simulink model "final_model"  (R2023b)
settings: Solver=VariableStepAuto  StartTime=0.0  StopTime=200  RelTol=1e-3
(part 3 of 3)

== system final_model/40g ==
  " u(t)" : Inport
  p(t) : Inport  Port=2
  Constant : Constant  Value=p1*Gb
  Constant1 : Constant  Value=p1
  Gain : Gain  Gain=1/V
  Gain1 : Gain  Gain=n
  Gain2 : Gain  Gain=p3
  Gain3 : Gain  Gain=-p2
  Gain4 : Gain  Gain=1/V
  Integrator : Integrator
  Integrator1 : Integrator
  Integrator2 : Integrator  InitialCondition=G0
  Product : Product
  Sum : Sum  Inputs=|+-
  Sum1 : Sum  Inputs=|++
  Sum2 : Sum  Inputs=|++-
  Sum3 : Sum  Inputs=|++
  " G(t)" : Outport
  X(t) : Outport  Port=2
  I(t) : Outport  Port=3
  wires:
  " u(t)"/1 -> Gain/1
  Gain/1 -> Sum/1
  Sum/1 -> Integrator/1
  Integrator/1 -> Gain2/1, I(t)/1, Gain1/1
  Gain1/1 -> Sum/2
  Gain2/1 -> Sum1/1
  Gain3/1 -> Sum1/2
  Integrator1/1 -> Gain3/1, Sum3/2, X(t)/1
  p(t)/1 -> Gain4/1
  Gain4/1 -> Sum2/1
  Constant/1 -> Sum2/2
  Constant1/1 -> Sum3/1
  Sum2/1 -> Integrator2/1
  Product/1 -> Sum2/3
  Sum3/1 -> Product/2
  Integrator2/1 -> Product/1, " G(t)"/1
  Sum1/1 -> Integrator1/1

== system final_model/40g.1 ==
  " u(t)" : Inport
  p(t) : Inport  Port=2
  Constant : Constant  Value=p1*Gb
  Constant1 : Constant  Value=p1
  Gain : Gain  Gain=1/V
  Gain1 : Gain  Gain=n
  Gain2 : Gain  Gain=p3
  Gain3 : Gain  Gain=-p2
  Gain4 : Gain  Gain=1/V
  Integrator : Integrator
  Integrator1 : Integrator
  Integrator2 : Integrator  InitialCondition=G0
  Product : Product
  Sum : Sum  Inputs=|+-
  Sum1 : Sum  Inputs=|++
  Sum2 : Sum  Inputs=|++-
  Sum3 : Sum  Inputs=|++
  " G(t)" : Outport
  X(t) : Outport  Port=2
  I(t) : Outport  Port=3
  wires:
  " u(t)"/1 -> Gain/1
  Gain/1 -> Sum/1
  Sum/1 -> Integrator/1
  Integrator/1 -> Gain2/1, I(t)/1, Gain1/1
  Gain1/1 -> Sum/2
  Gain2/1 -> Sum1/1
  Gain3/1 -> Sum1/2
  Integrator1/1 -> Gain3/1, Sum3/2, X(t)/1
  p(t)/1 -> Gain4/1
  Gain4/1 -> Sum2/1
  Constant/1 -> Sum2/2
  Constant1/1 -> Sum3/1
  Sum2/1 -> Integrator2/1
  Product/1 -> Sum2/3
  Sum3/1 -> Product/2
  Integrator2/1 -> Product/1, " G(t)"/1
  Sum1/1 -> Integrator1/1

== system final_model/40g1 ==
  " u(t)" : Inport
  p(t) : Inport  Port=2
  Constant : Constant  Value=p1*Gb
  Constant1 : Constant  Value=p1
  Gain : Gain  Gain=1/V
  Gain1 : Gain  Gain=n
  Gain2 : Gain  Gain=p3
  Gain3 : Gain  Gain=-p2
  Gain4 : Gain  Gain=1/V
  Integrator : Integrator
  Integrator1 : Integrator
  Integrator2 : Integrator  InitialCondition=G0
  Product : Product
  Sum : Sum  Inputs=|+-
  Sum1 : Sum  Inputs=|++
  Sum2 : Sum  Inputs=|++-
  Sum3 : Sum  Inputs=|++
  " G(t)" : Outport
  X(t) : Outport  Port=2
  I(t) : Outport  Port=3
  wires:
  " u(t)"/1 -> Gain/1
  Gain/1 -> Sum/1
  Sum/1 -> Integrator/1
  Integrator/1 -> Gain2/1, I(t)/1, Gain1/1
  Gain1/1 -> Sum/2
  Gain2/1 -> Sum1/1
  Gain3/1 -> Sum1/2
  Integrator1/1 -> Gain3/1, Sum3/2, X(t)/1
  p(t)/1 -> Gain4/1
  Gain4/1 -> Sum2/1
  Constant/1 -> Sum2/2
  Constant1/1 -> Sum3/1
  Sum2/1 -> Integrator2/1
  Product/1 -> Sum2/3
  Sum3/1 -> Product/2
  Integrator2/1 -> Product/1, " G(t)"/1
  Sum1/1 -> Integrator1/1

== system final_model/70.1g ==
  p(t) : Inport
  u(t) : Inport  Port=2
  Constant : Constant  Value=Gb
  Constant1 : Constant  Value=p1
  Gain : Gain  Gain=1/V
  Gain1 : Gain  Gain=p1
  Gain2 : Gain  Gain=p2
  Gain3 : Gain  Gain=1/V
  Gain4 : Gain  Gain=n
  Gain5 : Gain  Gain=p3
  Integrator : Integrator  InitialCondition=G0
  Integrator1 : Integrator
  Integrator2 : Integrator
  Product : Product
  Product1 : Product
  Sum : Sum  Inputs=|++--
  Sum1 : Sum  Inputs=|+-
  Sum2 : Sum  Inputs=|+-
  G(t) : Outport
  X(t) : Outport  Port=2
  I(t) : Outport  Port=3
  wires:
  Sum2/1 -> Integrator2/1
  Gain3/1 -> Sum2/1
  Sum1/1 -> Integrator1/1
  Integrator2/1 -> Gain4/1, I(t)/1, Gain5/1
  u(t)/1 -> Gain3/1
  Integrator1/1 -> Product1/2, X(t)/1, Gain2/1
  Product/1 -> Sum/2
  Integrator/1 -> G(t)/1, Gain1/1, Product1/1
  Gain5/1 -> Sum1/1
  Sum/1 -> Integrator/1
  Constant1/1 -> Product/2
  Constant/1 -> Product/1
  Gain4/1 -> Sum2/2
  Gain2/1 -> Sum1/2
  Product1/1 -> Sum/3
  Gain1/1 -> Sum/4
  p(t)/1 -> Gain/1
  Gain/1 -> Sum/1

== system final_model/70.1g1 ==
  p(t) : Inport
  u(t) : Inport  Port=2
  Constant : Constant  Value=Gb
  Constant1 : Constant  Value=p1
  Gain : Gain  Gain=1/V
  Gain1 : Gain  Gain=p1
  Gain2 : Gain  Gain=p2
  Gain3 : Gain  Gain=1/V
  Gain4 : Gain  Gain=n
  Gain5 : Gain  Gain=p3
  Integrator : Integrator  InitialCondition=G0
  Integrator1 : Integrator
  Integrator2 : Integrator
  Product : Product
  Product1 : Product
  Sum : Sum  Inputs=|++--
  Sum1 : Sum  Inputs=|+-
  Sum2 : Sum  Inputs=|+-
  G(t) : Outport
  X(t) : Outport  Port=2
  I(t) : Outport  Port=3
  wires:
  Sum2/1 -> Integrator2/1
  Gain3/1 -> Sum2/1
  Sum1/1 -> Integrator1/1
  Integrator2/1 -> Gain4/1, I(t)/1, Gain5/1
  u(t)/1 -> Gain3/1
  Integrator1/1 -> Product1/2, X(t)/1, Gain2/1
  Product/1 -> Sum/2
  Integrator/1 -> G(t)/1, Gain1/1, Product1/1
  Gain5/1 -> Sum1/1
  Sum/1 -> Integrator/1
  Constant1/1 -> Product/2
  Constant/1 -> Product/1
  Gain4/1 -> Sum2/2
  Gain2/1 -> Sum1/2
  Product1/1 -> Sum/3
  Gain1/1 -> Sum/4
  p(t)/1 -> Gain/1
  Gain/1 -> Sum/1

== system final_model/70g ==
  " u(t)" : Inport
  p(t) : Inport  Port=2
  Constant : Constant  Value=p1*Gb
  Constant1 : Constant  Value=p1
  Gain : Gain  Gain=1/V
  Gain1 : Gain  Gain=n
  Gain2 : Gain  Gain=p3
  Gain3 : Gain  Gain=-p2
  Gain4 : Gain  Gain=1/V
  Integrator : Integrator
  Integrator1 : Integrator
  Integrator2 : Integrator  InitialCondition=G0
  Product : Product
  Sum : Sum  Inputs=|+-
  Sum1 : Sum  Inputs=|++
  Sum2 : Sum  Inputs=|++-
  Sum3 : Sum  Inputs=|++
  " G(t)" : Outport
  X(t) : Outport  Port=2
  I(t) : Outport  Port=3
  wires:
  " u(t)"/1 -> Gain/1
  Gain/1 -> Sum/1
  Sum/1 -> Integrator/1
  Integrator/1 -> Gain2/1, I(t)/1, Gain1/1
  Gain1/1 -> Sum/2
  Gain2/1 -> Sum1/1
  Gain3/1 -> Sum1/2
  Integrator1/1 -> Gain3/1, Sum3/2, X(t)/1
  p(t)/1 -> Gain4/1
  Gain4/1 -> Sum2/1
  Constant/1 -> Sum2/2
  Constant1/1 -> Sum3/1
  Sum2/1 -> Integrator2/1
  Product/1 -> Sum2/3
  Sum3/1 -> Product/2
  Integrator2/1 -> Product/1, " G(t)"/1
  Sum1/1 -> Integrator1/1

== system final_model/70g.1 ==
  " u(t)" : Inport
  p(t) : Inport  Port=2
  Constant : Constant  Value=p1*Gb
  Constant1 : Constant  Value=p1
  Gain : Gain  Gain=1/V
  Gain1 : Gain  Gain=n
  Gain2 : Gain  Gain=p3
  Gain3 : Gain  Gain=-p2
  Gain4 : Gain  Gain=1/V
  Integrator : Integrator
  Integrator1 : Integrator
  Integrator2 : Integrator  InitialCondition=G0
  Product : Product
  Sum : Sum  Inputs=|+-
  Sum1 : Sum  Inputs=|++
  Sum2 : Sum  Inputs=|++-
  Sum3 : Sum  Inputs=|++
  " G(t)" : Outport
  X(t) : Outport  Port=2
  I(t) : Outport  Port=3
  wires:
  " u(t)"/1 -> Gain/1
  Gain/1 -> Sum/1
  Sum/1 -> Integrator/1
  Integrator/1 -> Gain2/1, I(t)/1, Gain1/1
  Gain1/1 -> Sum/2
  Gain2/1 -> Sum1/1
  Gain3/1 -> Sum1/2
  Integrator1/1 -> Gain3/1, Sum3/2, X(t)/1
  p(t)/1 -> Gain4/1
  Gain4/1 -> Sum2/1
  Constant/1 -> Sum2/2
  Constant1/1 -> Sum3/1
  Sum2/1 -> Integrator2/1
  Product/1 -> Sum2/3
  Sum3/1 -> Product/2
  Integrator2/1 -> Product/1, " G(t)"/1
  Sum1/1 -> Integrator1/1

== system final_model/70g1 ==
  " u(t)" : Inport
  p(t) : Inport  Port=2
  Constant : Constant  Value=p1*Gb
  Constant1 : Constant  Value=p1
  Gain : Gain  Gain=1/V
  Gain1 : Gain  Gain=n
  Gain2 : Gain  Gain=p3
  Gain3 : Gain  Gain=-p2
  Gain4 : Gain  Gain=1/V
  Integrator : Integrator
  Integrator1 : Integrator
  Integrator2 : Integrator  InitialCondition=G0
  Product : Product
  Sum : Sum  Inputs=|+-
  Sum1 : Sum  Inputs=|++
  Sum2 : Sum  Inputs=|++-
  Sum3 : Sum  Inputs=|++
  " G(t)" : Outport
  X(t) : Outport  Port=2
  I(t) : Outport  Port=3
  wires:
  " u(t)"/1 -> Gain/1
  Gain/1 -> Sum/1
  Sum/1 -> Integrator/1
  Integrator/1 -> Gain2/1, I(t)/1, Gain1/1
  Gain1/1 -> Sum/2
  Gain2/1 -> Sum1/1
  Gain3/1 -> Sum1/2
  Integrator1/1 -> Gain3/1, Sum3/2, X(t)/1
  p(t)/1 -> Gain4/1
  Gain4/1 -> Sum2/1
  Constant/1 -> Sum2/2
  Constant1/1 -> Sum3/1
  Sum2/1 -> Integrator2/1
  Product/1 -> Sum2/3
  Sum3/1 -> Product/2
  Integrator2/1 -> Product/1, " G(t)"/1
  Sum1/1 -> Integrator1/1

== system final_model/DG 100g ==
  " u(t)" : Inport
  p(t) : Inport  Port=2
  Constant : Constant  Value=p1*Gb
  Constant1 : Constant  Value=p1
  Gain : Gain  Gain=1/V
  Gain1 : Gain  Gain=n
  Gain2 : Gain  Gain=p3
  Gain3 : Gain  Gain=-p2
  Gain4 : Gain  Gain=1/V
  Integrator : Integrator
  Integrator1 : Integrator
  Integrator2 : Integrator  InitialCondition=G0
  Product : Product
  Sum : Sum  Inputs=|+-
  Sum1 : Sum  Inputs=|++
  Sum2 : Sum  Inputs=|++-
  Sum3 : Sum  Inputs=|++
  " G(t)" : Outport
  X(t) : Outport  Port=2
  I(t) : Outport  Port=3
  wires:
  " u(t)"/1 -> Gain/1
  Gain/1 -> Sum/1
  Sum/1 -> Integrator/1
  Integrator/1 -> Gain2/1, I(t)/1, Gain1/1
  Gain1/1 -> Sum/2
  Gain2/1 -> Sum1/1
  Gain3/1 -> Sum1/2
  Integrator1/1 -> Gain3/1, Sum3/2, X(t)/1
  p(t)/1 -> Gain4/1
  Gain4/1 -> Sum2/1
  Constant/1 -> Sum2/2
  Constant1/1 -> Sum3/1
  Sum2/1 -> Integrator2/1
  Product/1 -> Sum2/3
  Sum3/1 -> Product/2
  Integrator2/1 -> Product/1, " G(t)"/1
  Sum1/1 -> Integrator1/1

== system final_model/DG 10g ==
  " u(t)" : Inport
  p(t) : Inport  Port=2
  Constant : Constant  Value=p1*Gb
  Constant1 : Constant  Value=p1
  Gain : Gain  Gain=1/V
  Gain1 : Gain  Gain=n
  Gain2 : Gain  Gain=p3
  Gain3 : Gain  Gain=-p2
  Gain4 : Gain  Gain=1/V
  Integrator : Integrator
  Integrator1 : Integrator
  Integrator2 : Integrator  InitialCondition=G0
  Product : Product
  Sum : Sum  Inputs=|+-
  Sum1 : Sum  Inputs=|++
  Sum2 : Sum  Inputs=|++-
  Sum3 : Sum  Inputs=|++
  " G(t)" : Outport
  X(t) : Outport  Port=2
  I(t) : Outport  Port=3
  wires:
  " u(t)"/1 -> Gain/1
  Gain/1 -> Sum/1
  Sum/1 -> Integrator/1
  Integrator/1 -> Gain2/1, I(t)/1, Gain1/1
  Gain1/1 -> Sum/2
  Gain2/1 -> Sum1/1
  Gain3/1 -> Sum1/2
  Integrator1/1 -> Gain3/1, Sum3/2, X(t)/1
  p(t)/1 -> Gain4/1
  Gain4/1 -> Sum2/1
  Constant/1 -> Sum2/2
  Constant1/1 -> Sum3/1
  Sum2/1 -> Integrator2/1
  Product/1 -> Sum2/3
  Sum3/1 -> Product/2
  Integrator2/1 -> Product/1, " G(t)"/1
  Sum1/1 -> Integrator1/1

== system final_model/DG 40g ==
  " u(t)" : Inport
  p(t) : Inport  Port=2
  Constant : Constant  Value=p1*Gb
  Constant1 : Constant  Value=p1
  Gain : Gain  Gain=1/V
  Gain1 : Gain  Gain=n
  Gain2 : Gain  Gain=p3
  Gain3 : Gain  Gain=-p2
  Gain4 : Gain  Gain=1/V
  Integrator : Integrator
  Integrator1 : Integrator
  Integrator2 : Integrator  InitialCondition=G0
  Product : Product
  Sum : Sum  Inputs=|+-
  Sum1 : Sum  Inputs=|++
  Sum2 : Sum  Inputs=|++-
  Sum3 : Sum  Inputs=|++
  " G(t)" : Outport
  X(t) : Outport  Port=2
  I(t) : Outport  Port=3
  wires:
  " u(t)"/1 -> Gain/1
  Gain/1 -> Sum/1
  Sum/1 -> Integrator/1
  Integrator/1 -> Gain2/1, I(t)/1, Gain1/1
  Gain1/1 -> Sum/2
  Gain2/1 -> Sum1/1
  Gain3/1 -> Sum1/2
  Integrator1/1 -> Gain3/1, Sum3/2, X(t)/1
  p(t)/1 -> Gain4/1
  Gain4/1 -> Sum2/1
  Constant/1 -> Sum2/2
  Constant1/1 -> Sum3/1
  Sum2/1 -> Integrator2/1
  Product/1 -> Sum2/3
  Sum3/1 -> Product/2
  Integrator2/1 -> Product/1, " G(t)"/1
  Sum1/1 -> Integrator1/1

== system final_model/DG 70g ==
  " u(t)" : Inport
  p(t) : Inport  Port=2
  Constant : Constant  Value=p1*Gb
  Constant1 : Constant  Value=p1
  Gain : Gain  Gain=1/V
  Gain1 : Gain  Gain=n
  Gain2 : Gain  Gain=p3
  Gain3 : Gain  Gain=-p2
  Gain4 : Gain  Gain=1/V
  Integrator : Integrator
  Integrator1 : Integrator
  Integrator2 : Integrator  InitialCondition=G0
  Product : Product
  Sum : Sum  Inputs=|+-
  Sum1 : Sum  Inputs=|++
  Sum2 : Sum  Inputs=|++-
  Sum3 : Sum  Inputs=|++
  " G(t)" : Outport
  X(t) : Outport  Port=2
  I(t) : Outport  Port=3
  wires:
  " u(t)"/1 -> Gain/1
  Gain/1 -> Sum/1
  Sum/1 -> Integrator/1
  Integrator/1 -> Gain2/1, I(t)/1, Gain1/1
  Gain1/1 -> Sum/2
  Gain2/1 -> Sum1/1
  Gain3/1 -> Sum1/2
  Integrator1/1 -> Gain3/1, Sum3/2, X(t)/1
  p(t)/1 -> Gain4/1
  Gain4/1 -> Sum2/1
  Constant/1 -> Sum2/2
  Constant1/1 -> Sum3/1
  Sum2/1 -> Integrator2/1
  Product/1 -> Sum2/3
  Sum3/1 -> Product/2
  Integrator2/1 -> Product/1, " G(t)"/1
  Sum1/1 -> Integrator1/1

== system final_model/model liniar1 ==
  p(t) : Inport
  u(t) : Inport  Port=2
  Constant : Constant  Value=Gb
  Gain : Gain  Gain=1/V
  Gain1 : Gain  Gain=p1
  Gain2 : Gain  Gain=p2
  Gain3 : Gain  Gain=1/V
  Gain4 : Gain  Gain=n
  Gain5 : Gain  Gain=p3
  Integrator : Integrator  InitialCondition=G0
  Integrator1 : Integrator
  Integrator2 : Integrator
  Product : Product
  Product1 : Product
  Sum : Sum  Inputs=|+---
  Sum1 : Sum  Inputs=|+-
  Sum2 : Sum  Inputs=|+-
  Xb : Constant  Value=Xb
  G(t) : Outport
  X(t) : Outport  Port=2
  I(t) : Outport  Port=3
  wires:
  p(t)/1 -> Gain/1
  Gain/1 -> Sum/1
  Constant/1 -> Product/1
  Product/1 -> Sum/2
  Sum/1 -> Integrator/1
  Integrator/1 -> Gain1/1, Product1/1, G(t)/1
  Xb/1 -> Product1/2
  Product1/1 -> Sum/3
  Gain1/1 -> Sum/4
  Integrator1/1 -> Product/2, X(t)/1, Gain2/1
  Gain2/1 -> Sum1/2
  Integrator2/1 -> Gain4/1, I(t)/1, Gain5/1
  Sum2/1 -> Integrator2/1
  Gain5/1 -> Sum1/1
  Gain4/1 -> Sum2/2
  u(t)/1 -> Gain3/1
  Gain3/1 -> Sum2/1
  Sum1/1 -> Integrator1/1

== system final_model/model liniar2 ==
  p(t) : Inport
  u(t) : Inport  Port=2
  Constant : Constant  Value=Gb
  Gain : Gain  Gain=1/V
  Gain1 : Gain  Gain=p1
  Gain2 : Gain  Gain=p2
  Gain3 : Gain  Gain=1/V
  Gain4 : Gain  Gain=n
  Gain5 : Gain  Gain=p3
  Integrator : Integrator  InitialCondition=G0
  Integrator1 : Integrator
  Integrator2 : Integrator
  Product : Product
  Product1 : Product
  Sum : Sum  Inputs=|+---
  Sum1 : Sum  Inputs=|+-
  Sum2 : Sum  Inputs=|+-
  Xb : Constant  Value=Xb
  G(t) : Outport
  X(t) : Outport  Port=2
  I(t) : Outport  Port=3
  wires:
  p(t)/1 -> Gain/1
  Gain/1 -> Sum/1
  Constant/1 -> Product/1
  Product/1 -> Sum/2
  Sum/1 -> Integrator/1
  Integrator/1 -> Gain1/1, Product1/1, G(t)/1
  Xb/1 -> Product1/2
  Product1/1 -> Sum/3
  Gain1/1 -> Sum/4
  Integrator1/1 -> Product/2, X(t)/1, Gain2/1
  Gain2/1 -> Sum1/2
  Integrator2/1 -> Gain4/1, I(t)/1, Gain5/1
  Sum2/1 -> Integrator2/1
  Gain5/1 -> Sum1/1
  Gain4/1 -> Sum2/2
  u(t)/1 -> Gain3/1
  Gain3/1 -> Sum2/1
  Sum1/1 -> Integrator1/1

== system final_model/model liniar3 ==
  p(t) : Inport
  u(t) : Inport  Port=2
  Constant : Constant  Value=Gb
  Gain : Gain  Gain=1/V
  Gain1 : Gain  Gain=p1
  Gain2 : Gain  Gain=p2
  Gain3 : Gain  Gain=1/V
  Gain4 : Gain  Gain=n
  Gain5 : Gain  Gain=p3
  Integrator : Integrator  InitialCondition=G0
  Integrator1 : Integrator
  Integrator2 : Integrator
  Product : Product
  Product1 : Product
  Sum : Sum  Inputs=|+---
  Sum1 : Sum  Inputs=|+-
  Sum2 : Sum  Inputs=|+-
  Xb : Constant  Value=Xb
  G(t) : Outport
  X(t) : Outport  Port=2
  I(t) : Outport  Port=3
  wires:
  p(t)/1 -> Gain/1
  Gain/1 -> Sum/1
  Constant/1 -> Product/1
  Product/1 -> Sum/2
  Sum/1 -> Integrator/1
  Integrator/1 -> Gain1/1, Product1/1, G(t)/1
  Xb/1 -> Product1/2
  Product1/1 -> Sum/3
  Gain1/1 -> Sum/4
  Integrator1/1 -> Product/2, X(t)/1, Gain2/1
  Gain2/1 -> Sum1/2
  Integrator2/1 -> Gain4/1, I(t)/1, Gain5/1
  Sum2/1 -> Integrator2/1
  Gain5/1 -> Sum1/1
  Gain4/1 -> Sum2/2
  u(t)/1 -> Gain3/1
  Gain3/1 -> Sum2/1
  Sum1/1 -> Integrator1/1

== system final_model/model liniar4 ==
  p(t) : Inport
  u(t) : Inport  Port=2
  Constant : Constant  Value=Gb
  Gain : Gain  Gain=1/V
  Gain1 : Gain  Gain=p1
  Gain2 : Gain  Gain=p2
  Gain3 : Gain  Gain=1/V
  Gain4 : Gain  Gain=n
  Gain5 : Gain  Gain=p3
  Integrator : Integrator  InitialCondition=G0
  Integrator1 : Integrator
  Integrator2 : Integrator
  Product : Product
  Product1 : Product
  Sum : Sum  Inputs=|+---
  Sum1 : Sum  Inputs=|+-
  Sum2 : Sum  Inputs=|+-
  Xb : Constant  Value=Xb
  G(t) : Outport
  X(t) : Outport  Port=2
  I(t) : Outport  Port=3
  wires:
  p(t)/1 -> Gain/1
  Gain/1 -> Sum/1
  Constant/1 -> Product/1
  Product/1 -> Sum/2
  Sum/1 -> Integrator/1
  Integrator/1 -> Gain1/1, Product1/1, G(t)/1
  Xb/1 -> Product1/2
  Product1/1 -> Sum/3
  Gain1/1 -> Sum/4
  Integrator1/1 -> Product/2, X(t)/1, Gain2/1
  Gain2/1 -> Sum1/2
  Integrator2/1 -> Gain4/1, I(t)/1, Gain5/1
  Sum2/1 -> Integrator2/1
  Gain5/1 -> Sum1/1
  Gain4/1 -> Sum2/2
  u(t)/1 -> Gain3/1
  Gain3/1 -> Sum2/1
  Sum1/1 -> Integrator1/1

== system final_model/model_neliniar1 ==
  p(t) : Inport
  u(t) : Inport  Port=2
  Constant : Constant  Value=Gb
  Constant1 : Constant  Value=p1
  Gain : Gain  Gain=1/V
  Gain1 : Gain  Gain=p1
  Gain2 : Gain  Gain=p2
  Gain3 : Gain  Gain=1/V
  Gain4 : Gain  Gain=n
  Gain5 : Gain  Gain=p3
  Integrator : Integrator  InitialCondition=G0
  Integrator1 : Integrator
  Integrator2 : Integrator
  Product : Product
  Product1 : Product
  Sum : Sum  Inputs=|++--
  Sum1 : Sum  Inputs=|+-
  Sum2 : Sum  Inputs=|+-
  G(t) : Outport
  X(t) : Outport  Port=2
  I(t) : Outport  Port=3
  wires:
  Sum2/1 -> Integrator2/1
  Gain3/1 -> Sum2/1
  Sum1/1 -> Integrator1/1
  Integrator2/1 -> Gain4/1, I(t)/1, Gain5/1
  u(t)/1 -> Gain3/1
  Integrator1/1 -> Product1/2, X(t)/1, Gain2/1
  Product/1 -> Sum/2
  Integrator/1 -> G(t)/1, Gain1/1, Product1/1
  Gain5/1 -> Sum1/1
  Sum/1 -> Integrator/1
  Constant1/1 -> Product/2
  Constant/1 -> Product/1
  Gain4/1 -> Sum2/2
  Gain2/1 -> Sum1/2
  Product1/1 -> Sum/3
  Gain1/1 -> Sum/4
  p(t)/1 -> Gain/1
  Gain/1 -> Sum/1

== system final_model/model_neliniar2 ==
  p(t) : Inport
  u(t) : Inport  Port=2
  Constant : Constant  Value=Gb
  Constant1 : Constant  Value=p1
  Gain : Gain  Gain=1/V
  Gain1 : Gain  Gain=p1
  Gain2 : Gain  Gain=p2
  Gain3 : Gain  Gain=1/V
  Gain4 : Gain  Gain=n
  Gain5 : Gain  Gain=p3
  Integrator : Integrator  InitialCondition=G0
  Integrator1 : Integrator
  Integrator2 : Integrator
  Product : Product
  Product1 : Product
  Sum : Sum  Inputs=|++--
  Sum1 : Sum  Inputs=|+-
  Sum2 : Sum  Inputs=|+-
  G(t) : Outport
  X(t) : Outport  Port=2
  I(t) : Outport  Port=3
  wires:
  Sum2/1 -> Integrator2/1
  Gain3/1 -> Sum2/1
  Sum1/1 -> Integrator1/1
  Integrator2/1 -> Gain4/1, I(t)/1, Gain5/1
  u(t)/1 -> Gain3/1
  Integrator1/1 -> Product1/2, X(t)/1, Gain2/1
  Product/1 -> Sum/2
  Integrator/1 -> G(t)/1, Gain1/1, Product1/1
  Gain5/1 -> Sum1/1
  Sum/1 -> Integrator/1
  Constant1/1 -> Product/2
  Constant/1 -> Product/1
  Gain4/1 -> Sum2/2
  Gain2/1 -> Sum1/2
  Product1/1 -> Sum/3
  Gain1/1 -> Sum/4
  p(t)/1 -> Gain/1
  Gain/1 -> Sum/1

== system final_model/model_neliniar3 ==
  p(t) : Inport
  u(t) : Inport  Port=2
  Constant : Constant  Value=Gb
  Constant1 : Constant  Value=p1
  Gain : Gain  Gain=1/V
  Gain1 : Gain  Gain=p1
  Gain2 : Gain  Gain=p2
  Gain3 : Gain  Gain=1/V
  Gain4 : Gain  Gain=n
  Gain5 : Gain  Gain=p3
  Integrator : Integrator  InitialCondition=G0
  Integrator1 : Integrator
  Integrator2 : Integrator
  Product : Product
  Product1 : Product
  Sum : Sum  Inputs=|++--
  Sum1 : Sum  Inputs=|+-
  Sum2 : Sum  Inputs=|+-
  G(t) : Outport
  X(t) : Outport  Port=2
  I(t) : Outport  Port=3
  wires:
  Sum2/1 -> Integrator2/1
  Gain3/1 -> Sum2/1
  Sum1/1 -> Integrator1/1
  Integrator2/1 -> Gain4/1, I(t)/1, Gain5/1
  u(t)/1 -> Gain3/1
  Integrator1/1 -> Product1/2, X(t)/1, Gain2/1
  Product/1 -> Sum/2
  Integrator/1 -> G(t)/1, Gain1/1, Product1/1
  Gain5/1 -> Sum1/1
  Sum/1 -> Integrator/1
  Constant1/1 -> Product/2
  Constant/1 -> Product/1
  Gain4/1 -> Sum2/2
  Gain2/1 -> Sum1/2
  Product1/1 -> Sum/3
  Gain1/1 -> Sum/4
  p(t)/1 -> Gain/1
  Gain/1 -> Sum/1

== system final_model/model_neliniar4 ==
  p(t) : Inport
  u(t) : Inport  Port=2
  Constant : Constant  Value=Gb
  Constant1 : Constant  Value=p1
  Gain : Gain  Gain=1/V
  Gain1 : Gain  Gain=p1
  Gain2 : Gain  Gain=p2
  Gain3 : Gain  Gain=1/V
  Gain4 : Gain  Gain=n
  Gain5 : Gain  Gain=p3
  Integrator : Integrator  InitialCondition=G0
  Integrator1 : Integrator
  Integrator2 : Integrator
  Product : Product
  Product1 : Product
  Sum : Sum  Inputs=|++--
  Sum1 : Sum  Inputs=|+-
  Sum2 : Sum  Inputs=|+-
  G(t) : Outport
  X(t) : Outport  Port=2
  I(t) : Outport  Port=3
  wires:
  Sum2/1 -> Integrator2/1
  Gain3/1 -> Sum2/1
  Sum1/1 -> Integrator1/1
  Integrator2/1 -> Gain4/1, I(t)/1, Gain5/1
  u(t)/1 -> Gain3/1
  Integrator1/1 -> Product1/2, X(t)/1, Gain2/1
  Product/1 -> Sum/2
  Integrator/1 -> G(t)/1, Gain1/1, Product1/1
  Gain5/1 -> Sum1/1
  Sum/1 -> Integrator/1
  Constant1/1 -> Product/2
  Constant/1 -> Product/1
  Gain4/1 -> Sum2/2
  Gain2/1 -> Sum1/2
  Product1/1 -> Sum/3
  Gain1/1 -> Sum/4
  p(t)/1 -> Gain/1
  Gain/1 -> Sum/1

== system final_model/perturbatie1 ==
  Clock : Clock
  Constant : Constant  Value=Dg
  Constant1 : Constant  Value=Ag
  Gain : Gain  Gain=-1/tg_max
  Gain1 : Gain  Gain=1/(tg_max*tg_max)
  Math Function : Math
  Product : Product  Inputs=4
  p(t) : Outport
  wires:
  Constant/1 -> Product/1
  Constant1/1 -> Product/2
  Clock/1 -> Gain/1, Product/3
  Gain/1 -> Math Function/1
  Math Function/1 -> Product/4
  Product/1 -> Gain1/1
  Gain1/1 -> p(t)/1

== system final_model/perturbatie10 ==
  Clock : Clock
  Constant : Constant  Value=Dg
  Constant1 : Constant  Value=Ag
  Gain : Gain  Gain=-1/tg_max
  Gain1 : Gain  Gain=1/(tg_max*tg_max)
  Math Function : Math
  Product : Product  Inputs=4
  p(t) : Outport
  wires:
  Constant/1 -> Product/1
  Constant1/1 -> Product/2
  Clock/1 -> Gain/1, Product/3
  Gain/1 -> Math Function/1
  Math Function/1 -> Product/4
  Product/1 -> Gain1/1
  Gain1/1 -> p(t)/1

== system final_model/perturbatie11 ==
  Clock : Clock
  Constant : Constant  Value=Dg
  Constant1 : Constant  Value=Ag
  Gain : Gain  Gain=-1/tg_max
  Gain1 : Gain  Gain=1/(tg_max*tg_max)
  Math Function : Math
  Product : Product  Inputs=4
  p(t) : Outport
  wires:
  Constant/1 -> Product/1
  Constant1/1 -> Product/2
  Clock/1 -> Gain/1, Product/3
  Gain/1 -> Math Function/1
  Math Function/1 -> Product/4
  Product/1 -> Gain1/1
  Gain1/1 -> p(t)/1

== system final_model/perturbatie12 ==
  Clock : Clock
  Constant : Constant  Value=Dg
  Constant1 : Constant  Value=Ag
  Gain : Gain  Gain=-1/tg_max
  Gain1 : Gain  Gain=1/(tg_max*tg_max)
  Math Function : Math
  Product : Product  Inputs=4
  p(t) : Outport
  wires:
  Constant/1 -> Product/1
  Constant1/1 -> Product/2
  Clock/1 -> Gain/1, Product/3
  Gain/1 -> Math Function/1
  Math Function/1 -> Product/4
  Product/1 -> Gain1/1
  Gain1/1 -> p(t)/1

== system final_model/perturbatie13 ==
  Clock : Clock
  Constant : Constant  Value=Dg
  Constant1 : Constant  Value=Ag
  Gain : Gain  Gain=-1/tg_max
  Gain1 : Gain  Gain=1/(tg_max*tg_max)
  Math Function : Math
  Product : Product  Inputs=4
  p(t) : Outport
  wires:
  Constant/1 -> Product/1
  Constant1/1 -> Product/2
  Clock/1 -> Gain/1, Product/3
  Gain/1 -> Math Function/1
  Math Function/1 -> Product/4
  Product/1 -> Gain1/1
  Gain1/1 -> p(t)/1

== system final_model/perturbatie15 ==
  Clock : Clock
  Constant : Constant  Value=Dg
  Constant1 : Constant  Value=Ag
  Gain : Gain  Gain=-1/tg_max
  Gain1 : Gain  Gain=1/(tg_max*tg_max)
  Math Function : Math
  Product : Product  Inputs=4
  p(t) : Outport
  wires:
  Constant/1 -> Product/1
  Constant1/1 -> Product/2
  Clock/1 -> Gain/1, Product/3
  Gain/1 -> Math Function/1
  Math Function/1 -> Product/4
  Product/1 -> Gain1/1
  Gain1/1 -> p(t)/1

== system final_model/perturbatie16 ==
  Clock : Clock
  Constant : Constant  Value=Dg
  Constant1 : Constant  Value=Ag
  Gain : Gain  Gain=-1/tg_max
  Gain1 : Gain  Gain=1/(tg_max*tg_max)
  Math Function : Math
  Product : Product  Inputs=4
  p(t) : Outport
  wires:
  Constant/1 -> Product/1
  Constant1/1 -> Product/2
  Clock/1 -> Gain/1, Product/3
  Gain/1 -> Math Function/1
  Math Function/1 -> Product/4
  Product/1 -> Gain1/1
  Gain1/1 -> p(t)/1

== system final_model/perturbatie17 ==
  Clock : Clock
  Constant : Constant  Value=Dg
  Constant1 : Constant  Value=Ag
  Gain : Gain  Gain=-1/tg_max
  Gain1 : Gain  Gain=1/(tg_max*tg_max)
  Math Function : Math
  Product : Product  Inputs=4
  p(t) : Outport
  wires:
  Constant/1 -> Product/1
  Constant1/1 -> Product/2
  Clock/1 -> Gain/1, Product/3
  Gain/1 -> Math Function/1
  Math Function/1 -> Product/4
  Product/1 -> Gain1/1
  Gain1/1 -> p(t)/1

== system final_model/perturbatie18 ==
  Clock : Clock
  Constant : Constant  Value=Dg
  Constant1 : Constant  Value=Ag
  Gain : Gain  Gain=-1/tg_max
  Gain1 : Gain  Gain=1/(tg_max*tg_max)
  Math Function : Math
  Product : Product  Inputs=4
  p(t) : Outport
  wires:
  Constant/1 -> Product/1
  Constant1/1 -> Product/2
  Clock/1 -> Gain/1, Product/3
  Gain/1 -> Math Function/1
  Math Function/1 -> Product/4
  Product/1 -> Gain1/1
  Gain1/1 -> p(t)/1

== system final_model/perturbatie19 ==
  Clock : Clock
  Constant : Constant  Value=Dg
  Constant1 : Constant  Value=Ag
  Gain : Gain  Gain=-1/tg_max
  Gain1 : Gain  Gain=1/(tg_max*tg_max)
  Math Function : Math
  Product : Product  Inputs=4
  p(t) : Outport
  wires:
  Constant/1 -> Product/1
  Constant1/1 -> Product/2
  Clock/1 -> Gain/1, Product/3
  Gain/1 -> Math Function/1
  Math Function/1 -> Product/4
  Product/1 -> Gain1/1
  Gain1/1 -> p(t)/1

== system final_model/perturbatie2 ==
  Clock : Clock
  Constant : Constant  Value=Dg
  Constant1 : Constant  Value=Ag
  Gain : Gain  Gain=-1/tg_max
  Gain1 : Gain  Gain=1/(tg_max*tg_max)
  Math Function : Math
  Product : Product  Inputs=4
  p(t) : Outport
  wires:
  Constant/1 -> Product/1
  Constant1/1 -> Product/2
  Clock/1 -> Gain/1, Product/3
  Gain/1 -> Math Function/1
  Math Function/1 -> Product/4
  Product/1 -> Gain1/1
  Gain1/1 -> p(t)/1

== system final_model/perturbatie20 ==
  Clock : Clock
  Constant : Constant  Value=Dg
  Constant1 : Constant  Value=Ag
  Gain : Gain  Gain=-1/tg_max
  Gain1 : Gain  Gain=1/(tg_max*tg_max)
  Math Function : Math
  Product : Product  Inputs=4
  p(t) : Outport
  wires:
  Constant/1 -> Product/1
  Constant1/1 -> Product/2
  Clock/1 -> Gain/1, Product/3
  Gain/1 -> Math Function/1
  Math Function/1 -> Product/4
  Product/1 -> Gain1/1
  Gain1/1 -> p(t)/1

== system final_model/perturbatie21 ==
  Clock : Clock
  Constant : Constant  Value=Dg
  Constant1 : Constant  Value=Ag
  Gain : Gain  Gain=-1/tg_max
  Gain1 : Gain  Gain=1/(tg_max*tg_max)
  Math Function : Math
  Product : Product  Inputs=4
  p(t) : Outport
  wires:
  Constant/1 -> Product/1
  Constant1/1 -> Product/2
  Clock/1 -> Gain/1, Product/3
  Gain/1 -> Math Function/1
  Math Function/1 -> Product/4
  Product/1 -> Gain1/1
  Gain1/1 -> p(t)/1

== system final_model/perturbatie22 ==
  Clock : Clock
  Constant : Constant  Value=Dg
  Constant1 : Constant  Value=Ag
  Gain : Gain  Gain=-1/tg_max
  Gain1 : Gain  Gain=1/(tg_max*tg_max)
  Math Function : Math
  Product : Product  Inputs=4
  p(t) : Outport
  wires:
  Constant/1 -> Product/1
  Constant1/1 -> Product/2
  Clock/1 -> Gain/1, Product/3
  Gain/1 -> Math Function/1
  Math Function/1 -> Product/4
  Product/1 -> Gain1/1
  Gain1/1 -> p(t)/1

== system final_model/perturbatie23 ==
  Clock : Clock
  Constant : Constant  Value=Dg
  Constant1 : Constant  Value=Ag
  Gain : Gain  Gain=-1/tg_max
  Gain1 : Gain  Gain=1/(tg_max*tg_max)
  Math Function : Math
  Product : Product  Inputs=4
  p(t) : Outport
  wires:
  Constant/1 -> Product/1
  Constant1/1 -> Product/2
  Clock/1 -> Gain/1, Product/3
  Gain/1 -> Math Function/1
  Math Function/1 -> Product/4
  Product/1 -> Gain1/1
  Gain1/1 -> p(t)/1

== system final_model/perturbatie24 ==
  Clock : Clock
  Constant : Constant  Value=Dg
  Constant1 : Constant  Value=Ag
  Gain : Gain  Gain=-1/tg_max
  Gain1 : Gain  Gain=1/(tg_max*tg_max)
  Math Function : Math
  Product : Product  Inputs=4
  p(t) : Outport
  wires:
  Constant/1 -> Product/1
  Constant1/1 -> Product/2
  Clock/1 -> Gain/1, Product/3
  Gain/1 -> Math Function/1
  Math Function/1 -> Product/4
  Product/1 -> Gain1/1
  Gain1/1 -> p(t)/1

== system final_model/perturbatie25 ==
  Clock : Clock
  Constant : Constant  Value=Dg
  Constant1 : Constant  Value=Ag
  Gain : Gain  Gain=-1/tg_max
  Gain1 : Gain  Gain=1/(tg_max*tg_max)
  Math Function : Math
  Product : Product  Inputs=4
  p(t) : Outport
  wires:
  Constant/1 -> Product/1
  Constant1/1 -> Product/2
  Clock/1 -> Gain/1, Product/3
  Gain/1 -> Math Function/1
  Math Function/1 -> Product/4
  Product/1 -> Gain1/1
  Gain1/1 -> p(t)/1

== system final_model/perturbatie29 ==
  Clock : Clock
  Constant : Constant  Value=Dg
  Constant1 : Constant  Value=Ag
  Gain : Gain  Gain=-1/tg_max
  Gain1 : Gain  Gain=1/(tg_max*tg_max)
  Math Function : Math
  Product : Product  Inputs=4
  p(t) : Outport
  wires:
  Constant/1 -> Product/1
  Constant1/1 -> Product/2
  Clock/1 -> Gain/1, Product/3
  Gain/1 -> Math Function/1
  Math Function/1 -> Product/4
  Product/1 -> Gain1/1
  Gain1/1 -> p(t)/1

== system final_model/perturbatie3 ==
  Clock : Clock
  Constant : Constant  Value=Dg
  Constant1 : Constant  Value=Ag
  Gain : Gain  Gain=-1/tg_max
  Gain1 : Gain  Gain=1/(tg_max*tg_max)
  Math Function : Math
  Product : Product  Inputs=4
  p(t) : Outport
  wires:
  Constant/1 -> Product/1
  Constant1/1 -> Product/2
  Clock/1 -> Gain/1, Product/3
  Gain/1 -> Math Function/1
  Math Function/1 -> Product/4
  Product/1 -> Gain1/1
  Gain1/1 -> p(t)/1

== system final_model/perturbatie30 ==
  Clock : Clock
  Constant : Constant  Value=Dg
  Constant1 : Constant  Value=Ag
  Gain : Gain  Gain=-1/tg_max
  Gain1 : Gain  Gain=1/(tg_max*tg_max)
  Math Function : Math
  Product : Product  Inputs=4
  p(t) : Outport
  wires:
  Constant/1 -> Product/1
  Constant1/1 -> Product/2
  Clock/1 -> Gain/1, Product/3
  Gain/1 -> Math Function/1
  Math Function/1 -> Product/4
  Product/1 -> Gain1/1
  Gain1/1 -> p(t)/1

== system final_model/perturbatie31 ==
  Clock : Clock
  Constant : Constant  Value=Dg
  Constant1 : Constant  Value=Ag
  Gain : Gain  Gain=-1/tg_max
  Gain1 : Gain  Gain=1/(tg_max*tg_max)
  Math Function : Math
  Product : Product  Inputs=4
  p(t) : Outport
  wires:
  Constant/1 -> Product/1
  Constant1/1 -> Product/2
  Clock/1 -> Gain/1, Product/3
  Gain/1 -> Math Function/1
  Math Function/1 -> Product/4
  Product/1 -> Gain1/1
  Gain1/1 -> p(t)/1

== system final_model/perturbatie36 ==
  Clock : Clock
  Constant : Constant  Value=Dg
  Constant1 : Constant  Value=Ag
  Gain : Gain  Gain=-1/tg_max
  Gain1 : Gain  Gain=1/(tg_max*tg_max)
  Math Function : Math
  Product : Product  Inputs=4
  p(t) : Outport
  wires:
  Constant/1 -> Product/1
  Constant1/1 -> Product/2
  Clock/1 -> Gain/1, Product/3
  Gain/1 -> Math Function/1
  Math Function/1 -> Product/4
  Product/1 -> Gain1/1
  Gain1/1 -> p(t)/1

== system final_model/perturbatie37 ==
  Clock : Clock
  Constant : Constant  Value=Dg
  Constant1 : Constant  Value=Ag
  Gain : Gain  Gain=-1/tg_max
  Gain1 : Gain  Gain=1/(tg_max*tg_max)
  Math Function : Math
  Product : Product  Inputs=4
  p(t) : Outport
  wires:
  Constant/1 -> Product/1
  Constant1/1 -> Product/2
  Clock/1 -> Gain/1, Product/3
  Gain/1 -> Math Function/1
  Math Function/1 -> Product/4
  Product/1 -> Gain1/1
  Gain1/1 -> p(t)/1

== system final_model/perturbatie38 ==
  Clock : Clock
  Constant : Constant  Value=Dg
  Constant1 : Constant  Value=Ag
  Gain : Gain  Gain=-1/tg_max
  Gain1 : Gain  Gain=1/(tg_max*tg_max)
  Math Function : Math
  Product : Product  Inputs=4
  p(t) : Outport
  wires:
  Constant/1 -> Product/1
  Constant1/1 -> Product/2
  Clock/1 -> Gain/1, Product/3
  Gain/1 -> Math Function/1
  Math Function/1 -> Product/4
  Product/1 -> Gain1/1
  Gain1/1 -> p(t)/1

== system final_model/perturbatie39 ==
  Clock : Clock
  Constant : Constant  Value=Dg
  Constant1 : Constant  Value=Ag
  Gain : Gain  Gain=-1/tg_max
  Gain1 : Gain  Gain=1/(tg_max*tg_max)
  Math Function : Math
  Product : Product  Inputs=4
  p(t) : Outport
  wires:
  Constant/1 -> Product/1
  Constant1/1 -> Product/2
  Clock/1 -> Gain/1, Product/3
  Gain/1 -> Math Function/1
  Math Function/1 -> Product/4
  Product/1 -> Gain1/1
  Gain1/1 -> p(t)/1

== system final_model/perturbatie4 ==
  Clock : Clock
  Constant : Constant  Value=Dg
  Constant1 : Constant  Value=Ag
  Gain : Gain  Gain=-1/tg_max
  Gain1 : Gain  Gain=1/(tg_max*tg_max)
  Math Function : Math
  Product : Product  Inputs=4
  p(t) : Outport
  wires:
  Constant/1 -> Product/1
  Constant1/1 -> Product/2
  Clock/1 -> Gain/1, Product/3
  Gain/1 -> Math Function/1
  Math Function/1 -> Product/4
  Product/1 -> Gain1/1
  Gain1/1 -> p(t)/1

== system final_model/perturbatie5 ==
  Clock : Clock
  Constant : Constant  Value=Dg
  Constant1 : Constant  Value=Ag
  Gain : Gain  Gain=-1/tg_max
  Gain1 : Gain  Gain=1/(tg_max*tg_max)
  Math Function : Math
  Product : Product  Inputs=4
  p(t) : Outport
  wires:
  Constant/1 -> Product/1
  Constant1/1 -> Product/2
  Clock/1 -> Gain/1, Product/3
  Gain/1 -> Math Function/1
  Math Function/1 -> Product/4
  Product/1 -> Gain1/1
  Gain1/1 -> p(t)/1

== system final_model/perturbatie6 ==
  Clock : Clock
  Constant : Constant  Value=Dg
  Constant1 : Constant  Value=Ag
  Gain : Gain  Gain=-1/tg_max
  Gain1 : Gain  Gain=1/(tg_max*tg_max)
  Math Function : Math
  Product : Product  Inputs=4
  p(t) : Outport
  wires:
  Constant/1 -> Product/1
  Constant1/1 -> Product/2
  Clock/1 -> Gain/1, Product/3
  Gain/1 -> Math Function/1
  Math Function/1 -> Product/4
  Product/1 -> Gain1/1
  Gain1/1 -> p(t)/1

== system final_model/perturbatie7 ==
  Clock : Clock
  Constant : Constant  Value=Dg
  Constant1 : Constant  Value=Ag
  Gain : Gain  Gain=-1/tg_max
  Gain1 : Gain  Gain=1/(tg_max*tg_max)
  Math Function : Math
  Product : Product  Inputs=4
  p(t) : Outport
  wires:
  Constant/1 -> Product/1
  Constant1/1 -> Product/2
  Clock/1 -> Gain/1, Product/3
  Gain/1 -> Math Function/1
  Math Function/1 -> Product/4
  Product/1 -> Gain1/1
  Gain1/1 -> p(t)/1

== system final_model/perturbatie8 ==
  Clock : Clock
  Constant : Constant  Value=Dg
  Constant1 : Constant  Value=Ag
  Gain : Gain  Gain=-1/tg_max
  Gain1 : Gain  Gain=1/(tg_max*tg_max)
  Math Function : Math
  Product : Product  Inputs=4
  p(t) : Outport
  wires:
  Constant/1 -> Product/1
  Constant1/1 -> Product/2
  Clock/1 -> Gain/1, Product/3
  Gain/1 -> Math Function/1
  Math Function/1 -> Product/4
  Product/1 -> Gain1/1
  Gain1/1 -> p(t)/1

== system final_model/perturbatie9 ==
  Clock : Clock
  Constant : Constant  Value=Dg
  Constant1 : Constant  Value=Ag
  Gain : Gain  Gain=-1/tg_max
  Gain1 : Gain  Gain=1/(tg_max*tg_max)
  Math Function : Math
  Product : Product  Inputs=4
  p(t) : Outport
  wires:
  Constant/1 -> Product/1
  Constant1/1 -> Product/2
  Clock/1 -> Gain/1, Product/3
  Gain/1 -> Math Function/1
  Math Function/1 -> Product/4
  Product/1 -> Gain1/1
  Gain1/1 -> p(t)/1
